simulink model "Problem_7"  (R2020a)
settings: Solver=VariableStepAuto  StartTime=0.0  StopTime=10.0  RelTol=1e-3
libraries: simulink x1
settings Model: Creator=Ganesh  LastModifiedBy=Ganesh

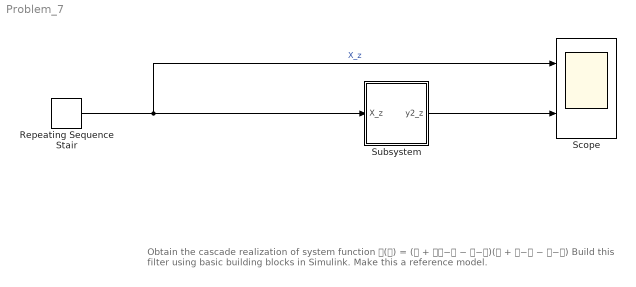
== system Problem_7 ==
  note: Obtain the cascade realization of system function
      | 𝐇(𝐳) = (𝟏 + 𝟐𝐳−𝟏 − 𝐳−𝟐)(𝟏 + 𝐳−𝟏 − 𝐳−𝟐)
      | Build this filter using basic building blocks in Simulink.
      | Make this a reference model.
  Repeating Sequence Stair : simulink/Sources/Repeating Sequence Stair  OutValues=[1 0 0 0 1 0 0 0 0 0 0 1].'  tsamp=-1  OutMin=[]  OutMax=[]  OutDataTypeStr=double  OutputDataTypeScalingMode=double  OutDataType=fixdt(0,8)  ConRadixGroup=Best Precision: Vector-wise  OutScaling=2^-12
  Scope : Scope  NumInputPorts=2
  Subsystem : Subsystem
  wires:
  Repeating Sequence Stair/1 -> Subsystem/1(X_z), Scope/1  "X_z"
  Subsystem/1(y2_z) -> Scope/2

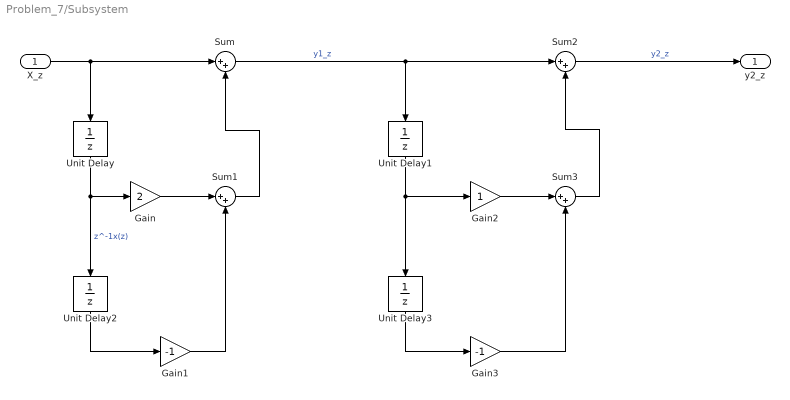
== system Problem_7/Subsystem ==
  X_z : Inport
  Gain : Gain  Gain=2
  Gain1 : Gain  Gain=-1
  Gain2 : Gain
  Gain3 : Gain  Gain=-1
  Sum{,1..3} (4 alike) : Sum  Inputs=|++
  Unit Delay{,1..3} (4 alike) : UnitDelay  SampleTime=-1  HasFrameUpgradeWarning=on
  y2_z : Outport
  wires:
  X_z/1 -> Unit Delay/1, Sum/1
  Unit Delay/1 -> Gain/1, Unit Delay2/1  "z^-1x(z)"
  Sum1/1 -> Sum/2
  Gain3/1 -> Sum3/2
  Unit Delay1/1 -> Gain2/1, Unit Delay3/1
  Unit Delay2/1 -> Gain1/1
  Gain1/1 -> Sum1/2
  Gain/1 -> Sum1/1
  Unit Delay3/1 -> Gain3/1
  Sum/1 -> Sum2/1, Unit Delay1/1  "y1_z"
  Sum3/1 -> Sum2/2
  Gain2/1 -> Sum3/1
  Sum2/1 -> y2_z/1  "y2_z"
